simulink model "ex1"  (R2024b)
settings: Solver=VariableStepAuto  StartTime=0.0  StopTime=5  RelTol=1e-3
values from neighbouring files (symbols this model uses):
  Kd = Kp*Td    [ex1_startup.m]
  Ki = Kp/Ti    [ex1_startup.m]
  Kp = delta_k*cos(delta_phi)    [ex1_startup.m]
  Kw = 5/(3/(d*w_gc))    [ex1_startup.m]
  Tl = 5/(2*w_gc)    [ex1_startup.m]
undefined symbols (not defined in the file or in its folder): plant, sIn
libraries: simulink x1
settings Model: Creator=Nihal  LastModifiedBy=Nihal

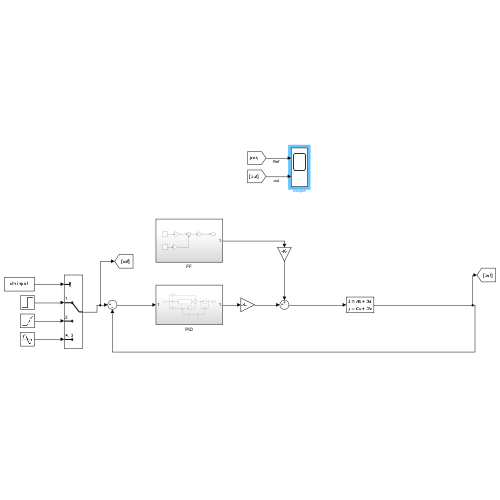
[thumbnail: Simulink's stored preview of the top-level diagram]
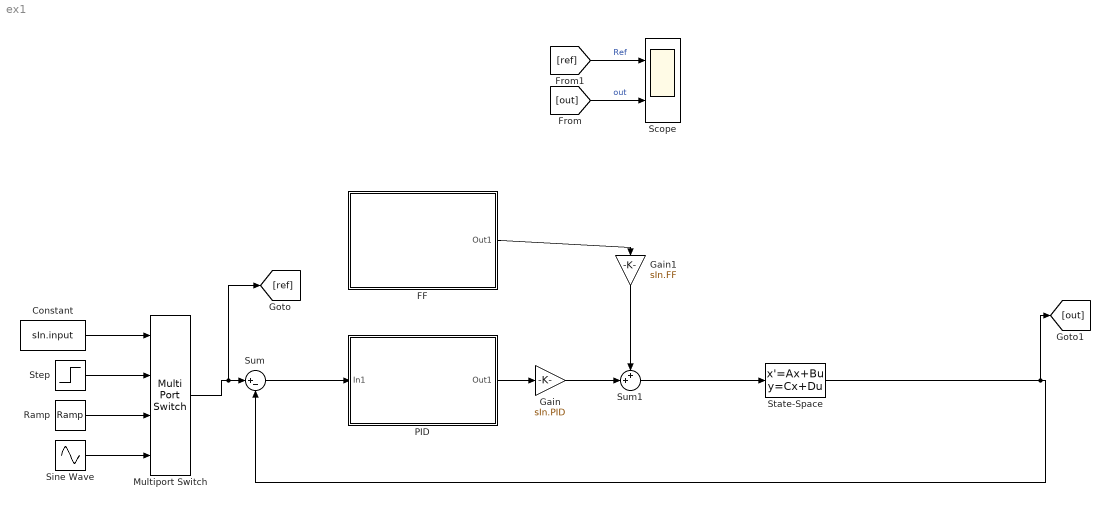
== system ex1 ==
  Constant : Constant  Value=sIn.input
  FF : Subsystem
  Gain : Gain  Gain=sIn.PID
  Gain1 : Gain  Gain=sIn.FF
  Multiport Switch : MultiPortSwitch  SaturateOnIntegerOverflow=off  InputSameDT=off
  PID : Subsystem
  Ramp : simulink/Sources/Ramp  slope=30  start=0  InitialOutput=0
  Scope : Scope  NumInputPorts=2
  Sine Wave : Sin  Frequency=10  SampleTime=0
  State-Space : StateSpace  A=plant.A  B=plant.B  C=plant.C  D=plant.D  InitialCondition=0
  Step : Step  Time=0  After=40  SampleTime=0
  Sum : Sum  Inputs=|+-
  Sum1 : Sum  Inputs=++|
  wires:
  Sum/1 -> PID/1(In1)
  State-Space/1 -> [out], Sum/2
  Ramp/1 -> Multiport Switch/3
  Step/1 -> Multiport Switch/2
  Multiport Switch/1 -> [ref], Sum/1
  Constant/1 -> Multiport Switch/1
  Sine Wave/1 -> Multiport Switch/4
  Sum1/1 -> State-Space/1
  PID/1(Out1) -> Gain/1
  Gain/1 -> Sum1/2
  FF/1(Out1) -> Gain1/1
  Gain1/1 -> Sum1/1
  [out] -> Scope/2  "out"
  [ref] -> Scope/1  "Ref"

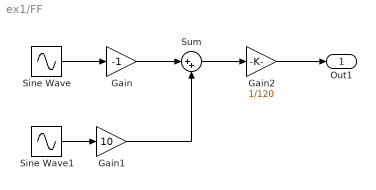
== system ex1/FF ==
  Gain : Gain  Gain=-1
  Gain1 : Gain  Gain=10
  Gain2 : Gain  Gain=1/120
  Sine Wave : Sin  Amplitude=100  Frequency=10  SampleTime=0
  Sine Wave1 : Sin  Amplitude=10  Frequency=10  Phase=pi/2  SampleTime=0
  Sum : Sum  Inputs=|++
  Out1 : Outport
  wires:
  Sine Wave/1 -> Gain/1
  Sine Wave1/1 -> Gain1/1
  Gain/1 -> Sum/1
  Gain1/1 -> Sum/2
  Sum/1 -> Gain2/1
  Gain2/1 -> Out1/1

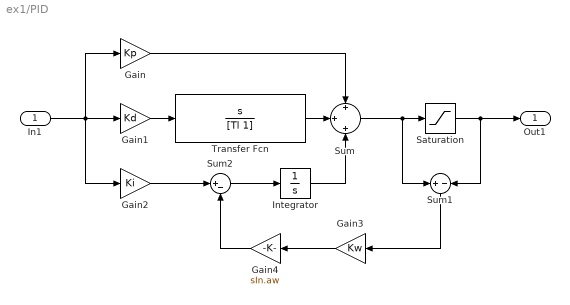
== system ex1/PID ==
  In1 : Inport
  Gain : Gain  Gain=Kp
  Gain1 : Gain  Gain=Kd
  Gain2 : Gain  Gain=Ki
  Gain3 : Gain  Gain=Kw
  Gain4 : Gain  Gain=sIn.aw
  Integrator : Integrator
  Saturation : Saturate  UpperLimit=10  LowerLimit=-10
  Sum : Sum  Inputs=+|+|+
  Sum1 : Sum  Inputs=+|-
  Sum2 : Sum  Inputs=|+-
  Transfer Fcn : TransferFcn  Numerator=[1 0]  Denominator=[Tl 1]
  Out1 : Outport
  wires:
  In1/1 -> Gain2/1, Gain1/1, Gain/1
  Integrator/1 -> Sum/3
  Gain/1 -> Sum/1
  Gain1/1 -> Transfer Fcn/1
  Transfer Fcn/1 -> Sum/2
  Sum/1 -> Sum1/1, Saturation/1
  Saturation/1 -> Sum1/2, Out1/1
  Sum1/1 -> Gain3/1
  Gain2/1 -> Sum2/1
  Sum2/1 -> Integrator/1
  Gain3/1 -> Gain4/1
  Gain4/1 -> Sum2/2
